simulink model "adc_interrupt_current_loop_triggered"  (R2023b)
settings: Solver=FixedStepDiscrete  StartTime=0  StopTime=0.02  FixedStep=1e-06  RelTol=1e-3
undefined symbols (not defined in the file or in its folder): DiscIntNeverNeededParam
libraries: simulink x2
settings Model: Creator=user  LastModifiedBy=user
settings HardwareCC: ProdBitPerLong=64  ProdHWDeviceType=Intel->x86-64 (Linux 64)  TargetBitPerLong=64  TargetBitPerPointer=64  TargetBitPerSizeT=64  TargetBitPerPtrDiffT=64  TargetLargestAtomicFloat=Float  TargetIntDivRoundTo=Zero  TargetEndianess=LittleEndian  TargetWordSize=64  TargetHWDeviceType=Intel->x86-64 (Linux 64)  ProdEqTarget=off
settings RTWCC: GenerateReport=on

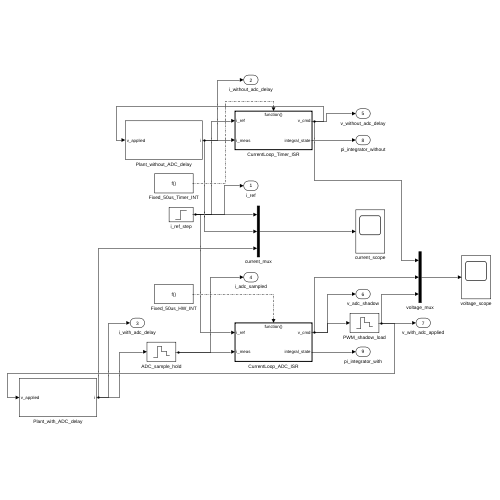
[thumbnail: Simulink's stored preview of the top-level diagram]
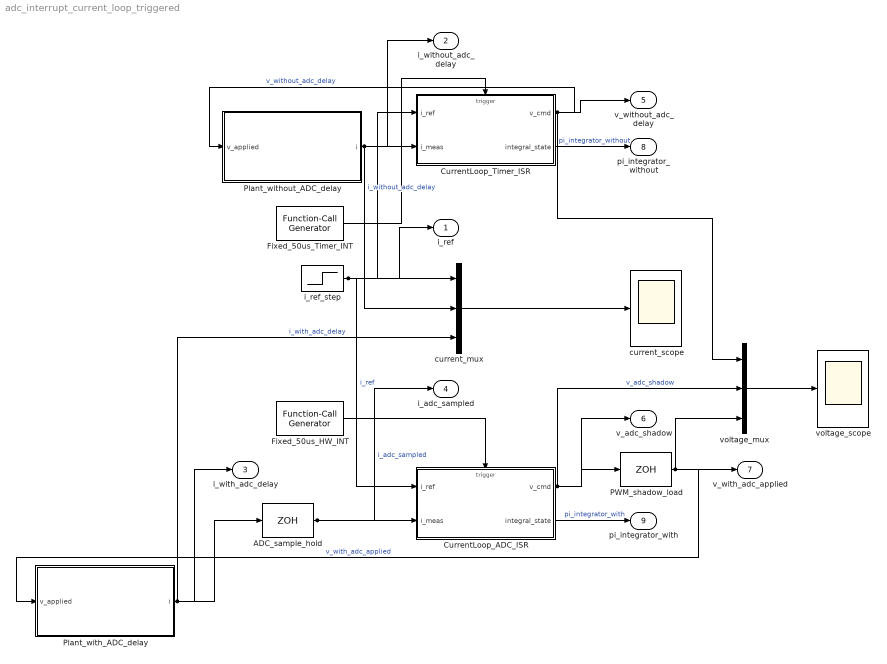
== system adc_interrupt_current_loop_triggered ==
  ADC_sample_hold : ZeroOrderHold  SampleTime=5e-05
  CurrentLoop_ADC_ISR : Subsystem  TreatAsAtomicUnit=on  RTWFcnName=current_loop_adc_isr  RTWFileName=current_loop_adc_isr
      settings: RTWFcnNameOpts=User specified  RTWFileNameOpts=User specified
  CurrentLoop_Timer_ISR : Subsystem  TreatAsAtomicUnit=on  RTWFcnName=current_loop_timer_isr  RTWFileName=current_loop_timer_isr
      settings: RTWFcnNameOpts=User specified  RTWFileNameOpts=User specified
  Fixed_50us_HW_INT : simulink/Ports & Subsystems/Function-Call Generator  sample_time=5e-05  numberOfIterations=1  DisallowWideOutput=off
  Fixed_50us_Timer_INT : simulink/Ports & Subsystems/Function-Call Generator  sample_time=5e-05  numberOfIterations=1  DisallowWideOutput=off
  PWM_shadow_load : ZeroOrderHold  SampleTime=5e-05
  Plant_with_ADC_delay : Subsystem
  Plant_without_ADC_delay : Subsystem
  current_mux : Mux  Inputs=3
  current_scope : Scope
  i_ref_step : Step  Time=0.002  After=10  SampleTime=1e-06
  voltage_mux : Mux  Inputs=3
  voltage_scope : Scope
  i_ref : Outport
  i_without_adc_delay : Outport  Port=2
  i_with_adc_delay : Outport  Port=3
  i_adc_sampled : Outport  Port=4
  v_without_adc_delay : Outport  Port=5
  v_adc_shadow : Outport  Port=6
  v_with_adc_applied : Outport  Port=7
  pi_integrator_without : Outport  Port=8
  pi_integrator_with : Outport  Port=9
  wires:
  voltage_mux/1 -> voltage_scope/1
  CurrentLoop_ADC_ISR/1(v_cmd) -> v_adc_shadow/1, PWM_shadow_load/1, voltage_mux/2  "v_adc_shadow"
  current_mux/1 -> current_scope/1
  CurrentLoop_Timer_ISR/2(integral_state) -> pi_integrator_without/1  "pi_integrator_without"
  ADC_sample_hold/1 -> i_adc_sampled/1, CurrentLoop_ADC_ISR/2(i_meas)  "i_adc_sampled"
  PWM_shadow_load/1 -> voltage_mux/3, v_with_adc_applied/1, Plant_with_ADC_delay/1(v_applied)  "v_with_adc_applied"
  Fixed_50us_HW_INT/1 -> CurrentLoop_ADC_ISR/Trigger
  i_ref_step/1 -> current_mux/1, CurrentLoop_Timer_ISR/1(i_ref), i_ref/1, CurrentLoop_ADC_ISR/1(i_ref)  "i_ref"
  Fixed_50us_Timer_INT/1 -> CurrentLoop_Timer_ISR/Trigger
  CurrentLoop_Timer_ISR/1(v_cmd) -> v_without_adc_delay/1, voltage_mux/1, Plant_without_ADC_delay/1(v_applied)  "v_without_adc_delay"
  Plant_without_ADC_delay/1(i) -> current_mux/2, i_without_adc_delay/1, CurrentLoop_Timer_ISR/2(i_meas)  "i_without_adc_delay"
  CurrentLoop_ADC_ISR/2(integral_state) -> pi_integrator_with/1  "pi_integrator_with"
  Plant_with_ADC_delay/1(i) -> i_with_adc_delay/1, ADC_sample_hold/1, current_mux/3  "i_with_adc_delay"

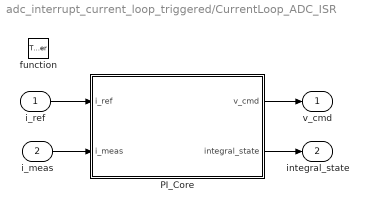
== system adc_interrupt_current_loop_triggered/CurrentLoop_ADC_ISR ==
  i_ref : Inport
  i_meas : Inport  Port=2
  function : TriggerPort  TriggerType=function-call  VariantControl=(inherit)
  PI_Core : MATLAB Function  TreatAsAtomicUnit=on
  v_cmd : Outport
  integral_state : Outport  Port=2
  wires:
  PI_Core/1(v_cmd) -> v_cmd/1
  PI_Core/2(integral_state) -> integral_state/1
  i_meas/1 -> PI_Core/2(i_meas)
  i_ref/1 -> PI_Core/1(i_ref)

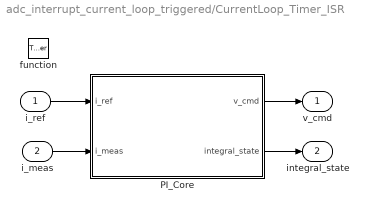
== system adc_interrupt_current_loop_triggered/CurrentLoop_Timer_ISR ==
  i_ref : Inport
  i_meas : Inport  Port=2
  function : TriggerPort  TriggerType=function-call  VariantControl=(inherit)
  PI_Core : MATLAB Function  TreatAsAtomicUnit=on
  v_cmd : Outport
  integral_state : Outport  Port=2
  wires:
  PI_Core/1(v_cmd) -> v_cmd/1
  i_meas/1 -> PI_Core/2(i_meas)
  PI_Core/2(integral_state) -> integral_state/1
  i_ref/1 -> PI_Core/1(i_ref)

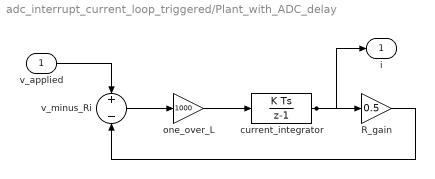
== system adc_interrupt_current_loop_triggered/Plant_with_ADC_delay ==
  v_applied : Inport
  R_gain : Gain  Gain=0.5
  current_integrator : DiscreteIntegrator  gainval=1  SampleTime=9.9999999999999995e-07  ICPrevOutput=DiscIntNeverNeededParam  ICPrevScaledInput=DiscIntNeverNeededParam
  one_over_L : Gain  Gain=1000
  v_minus_Ri : Sum  Inputs=+-
  i : Outport
  wires:
  R_gain/1 -> v_minus_Ri/2
  one_over_L/1 -> current_integrator/1
  current_integrator/1 -> R_gain/1, i/1
  v_minus_Ri/1 -> one_over_L/1
  v_applied/1 -> v_minus_Ri/1

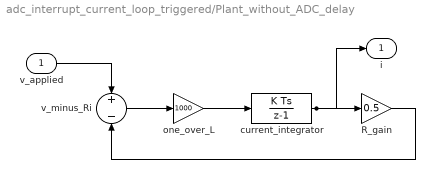
== system adc_interrupt_current_loop_triggered/Plant_without_ADC_delay ==
  v_applied : Inport
  R_gain : Gain  Gain=0.5
  current_integrator : DiscreteIntegrator  gainval=1  SampleTime=9.9999999999999995e-07  ICPrevOutput=DiscIntNeverNeededParam  ICPrevScaledInput=DiscIntNeverNeededParam
  one_over_L : Gain  Gain=1000
  v_minus_Ri : Sum  Inputs=+-
  i : Outport
  wires:
  R_gain/1 -> v_minus_Ri/2
  current_integrator/1 -> R_gain/1, i/1
  one_over_L/1 -> current_integrator/1
  v_minus_Ri/1 -> one_over_L/1
  v_applied/1 -> v_minus_Ri/1

== matlab function adc_interrupt_current_loop_triggered/CurrentLoop_Timer_ISR/PI_Core ==
  data: i_ref input; v_cmd output; i_meas input; integral_state output
function [v_cmd, integral_state] = fcn(i_ref, i_meas)
%#codegen
persistent integrator
if isempty(integrator)
    integrator = 0.0;
end
Ts = 5.0000000000000002e-05;
Kp = 5.026548245743669;
Ki = 2513.2741228718346;
V_limit = 24;
integrator_limit = 24;
e = i_ref - i_meas;
p_term = Kp * e;
integrator = integrator + Ki * Ts * e;
integrator = min(max(integrator, -integrator_limit), integrator_limit);
v_unsat = p_term + integrator;
v_cmd = min(max(v_unsat, -V_limit), V_limit);
if v_cmd ~= v_unsat
    integrator = v_cmd - p_term;
    integrator = min(max(integrator, -integrator_limit), integrator_limit);
end
integral_state = integrator;
end

== matlab function adc_interrupt_current_loop_triggered/CurrentLoop_ADC_ISR/PI_Core ==
  data: i_ref input; v_cmd output; i_meas input; integral_state output
function [v_cmd, integral_state] = fcn(i_ref, i_meas)
%#codegen
persistent integrator
if isempty(integrator)
    integrator = 0.0;
end
Ts = 5.0000000000000002e-05;
Kp = 5.026548245743669;
Ki = 2513.2741228718346;
V_limit = 24;
integrator_limit = 24;
e = i_ref - i_meas;
p_term = Kp * e;
integrator = integrator + Ki * Ts * e;
integrator = min(max(integrator, -integrator_limit), integrator_limit);
v_unsat = p_term + integrator;
v_cmd = min(max(v_unsat, -V_limit), V_limit);
if v_cmd ~= v_unsat
    integrator = v_cmd - p_term;
    integrator = min(max(integrator, -integrator_limit), integrator_limit);
end
integral_state = integrator;
end
